simulink model "Check_my_Aerodynamics_for_Mac"  (R2020b)
settings: Solver=FixedStepAuto  StartTime=0.0  StopTime=100  FixedStep=CNT_StepSize  RelTol=1e-3
undefined symbols (not defined in the file): CNT_StepSize
libraries: simulink x2
settings Model: Creator=NicolasS  LastModifiedBy=benjaminh

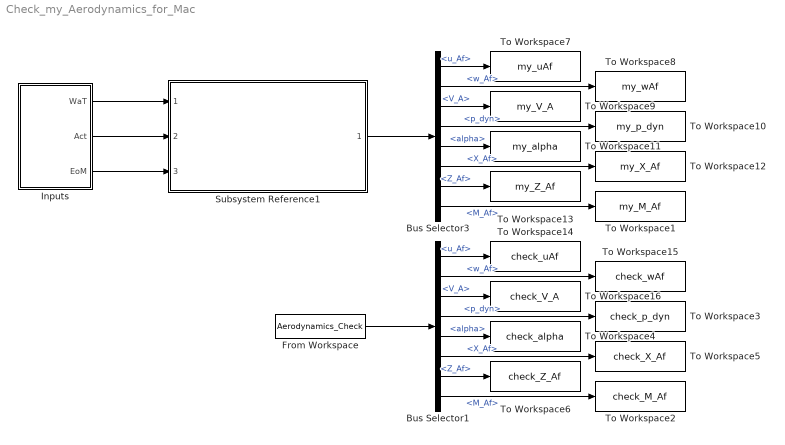
== system Check_my_Aerodynamics_for_Mac ==
  Bus Selector1 : BusSelector  OutputSignals=AirData.u_Af,AirData.w_Af,AirData.V_A,AirData.p_dyn,AirData.alpha,X_Af,Z_Af,M_Af
  Bus Selector3 : BusSelector  OutputSignals=AirData.u_Af,AirData.w_Af,AirData.V_A,AirData.p_dyn,AirData.alpha,X_Af,Z_Af,M_Af
  From Workspace : FromWorkspace  VariableName=Aerodynamics_Check  OutDataTypeStr=Bus: Aero  SampleTime=CNT_StepSize
  Inputs : Subsystem
  Subsystem Reference1 : Subsystem  ReferencedSubsystem=Aerodyn
  To Workspace1 : ToWorkspace  VariableName=my_M_Af  SaveFormat=Timeseries  SampleTime=-1
  To Workspace10 : ToWorkspace  VariableName=my_p_dyn  SaveFormat=Timeseries  SampleTime=-1
  To Workspace11 : ToWorkspace  VariableName=my_alpha  SaveFormat=Timeseries  SampleTime=-1
  To Workspace12 : ToWorkspace  VariableName=my_X_Af  SaveFormat=Timeseries  SampleTime=-1
  To Workspace13 : ToWorkspace  VariableName=my_Z_Af  SaveFormat=Timeseries  SampleTime=-1
  To Workspace14 : ToWorkspace  VariableName=check_uAf  SaveFormat=Timeseries  SampleTime=-1
  To Workspace15 : ToWorkspace  VariableName=check_wAf  SaveFormat=Timeseries  SampleTime=-1
  To Workspace16 : ToWorkspace  VariableName=check_V_A  SaveFormat=Timeseries  SampleTime=-1
  To Workspace2 : ToWorkspace  VariableName=check_M_Af  SaveFormat=Timeseries  SampleTime=-1
  To Workspace3 : ToWorkspace  VariableName=check_p_dyn  SaveFormat=Timeseries  SampleTime=-1
  To Workspace4 : ToWorkspace  VariableName=check_alpha  SaveFormat=Timeseries  SampleTime=-1
  To Workspace5 : ToWorkspace  VariableName=check_X_Af  SaveFormat=Timeseries  SampleTime=-1
  To Workspace6 : ToWorkspace  VariableName=check_Z_Af  SaveFormat=Timeseries  SampleTime=-1
  To Workspace7 : ToWorkspace  VariableName=my_uAf  SaveFormat=Timeseries  SampleTime=-1
  To Workspace8 : ToWorkspace  VariableName=my_wAf  SaveFormat=Timeseries  SampleTime=-1
  To Workspace9 : ToWorkspace  VariableName=my_V_A  SaveFormat=Timeseries  SampleTime=-1
  wires:
  Bus Selector3/7 -> To Workspace13/1  "<Z_Af>"
  Bus Selector3/2 -> To Workspace8/1  "<w_Af>"
  Bus Selector3/6 -> To Workspace12/1  "<X_Af>"
  Bus Selector3/3 -> To Workspace9/1  "<V_A>"
  Bus Selector3/1 -> To Workspace7/1  "<u_Af>"
  Bus Selector3/5 -> To Workspace11/1  "<alpha>"
  Bus Selector3/4 -> To Workspace10/1  "<p_dyn>"
  Subsystem Reference1/1 -> Bus Selector3/1
  Bus Selector3/8 -> To Workspace1/1  "<M_Af>"
  Bus Selector1/4 -> To Workspace3/1  "<p_dyn>"
  Bus Selector1/8 -> To Workspace2/1  "<M_Af>"
  Bus Selector1/7 -> To Workspace6/1  "<Z_Af>"
  Bus Selector1/5 -> To Workspace4/1  "<alpha>"
  Bus Selector1/1 -> To Workspace14/1  "<u_Af>"
  Bus Selector1/6 -> To Workspace5/1  "<X_Af>"
  Bus Selector1/2 -> To Workspace15/1  "<w_Af>"
  Bus Selector1/3 -> To Workspace16/1  "<V_A>"
  Inputs/2(Act) -> Subsystem Reference1/2
  Inputs/1(WaT) -> Subsystem Reference1/1
  Inputs/3(EoM) -> Subsystem Reference1/3
  From Workspace/1 -> Bus Selector1/1

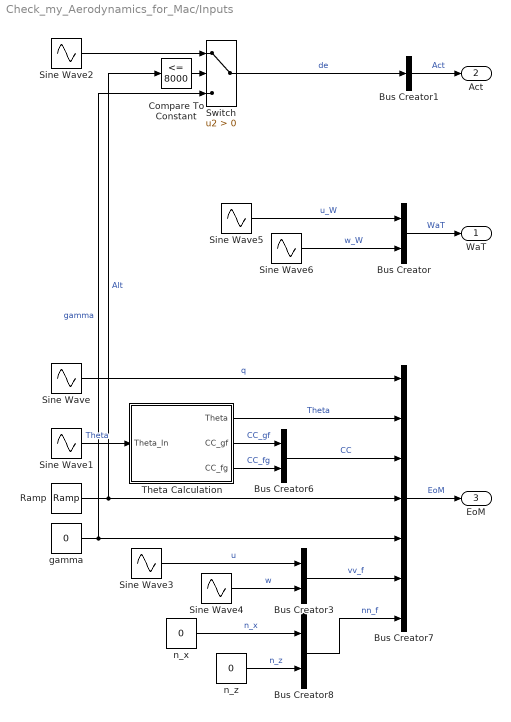
== system Check_my_Aerodynamics_for_Mac/Inputs ==
  Bus Creator : BusCreator  Inputs=2  OutDataTypeStr=Bus: WaT
  Bus Creator1 : BusCreator  Inputs=1  OutDataTypeStr=Bus: Act
  Bus Creator3 : BusCreator  Inputs=2  OutDataTypeStr=Bus: vv_f
  Bus Creator6 : BusCreator  Inputs=2  OutDataTypeStr=Bus: CC
  Bus Creator7 : BusCreator  Inputs=7  OutDataTypeStr=Bus: EoM
  Bus Creator8 : BusCreator  Inputs=2  OutDataTypeStr=Bus: nn_f
  Compare To Constant : simulink/Logic and Bit Operations/Compare To Constant  relop=<=  const=8000  OutDataTypeStr=boolean
  Ramp : simulink/Sources/Ramp  slope=-50  start=0  InitialOutput=10000
  Sine Wave : Sin  Amplitude=0.05  Frequency=0.9  SampleTime=CNT_StepSize
  Sine Wave1 : Sin  Amplitude=0.1  Frequency=0.1  Phase=-45  SampleTime=CNT_StepSize
  Sine Wave2 : Sin  Amplitude=0.03  Frequency=1.3  Phase=-67  SampleTime=CNT_StepSize
  Sine Wave3 : Sin  Amplitude=20  Bias=140  Frequency=0.1  Phase=34  SampleTime=CNT_StepSize
  Sine Wave4 : Sin  Amplitude=5  Bias=7  Frequency=0.24  SampleTime=CNT_StepSize
  Sine Wave5 : Sin  Amplitude=15  Frequency=2*pi/40  Phase=63  SampleTime=CNT_StepSize
  Sine Wave6 : Sin  Amplitude=5  Frequency=2*pi/40  Phase=-15  SampleTime=CNT_StepSize
  Switch : Switch  Criteria=u2 > Threshold
  Theta Calculation : MATLAB Function  TreatAsAtomicUnit=on
  gamma : Constant  Value=0  SampleTime=-1
  n_x : Constant  Value=0  SampleTime=-1
  n_z : Constant  Value=0  SampleTime=-1
  WaT : Outport  OutDataTypeStr=Bus: WaT
  Act : Outport  Port=2  OutDataTypeStr=Bus: Act
  EoM : Outport  Port=3  OutDataTypeStr=Bus: EoM
  wires:
  Bus Creator8/1 -> Bus Creator7/7  "nn_f"
  Sine Wave3/1 -> Bus Creator3/1  "u"
  n_x/1 -> Bus Creator8/1  "n_x"
  Bus Creator3/1 -> Bus Creator7/6  "vv_f"
  Sine Wave5/1 -> Bus Creator/1  "u_W"
  Theta Calculation/2(CC_gf) -> Bus Creator6/1  "CC_gf"
  Bus Creator/1 -> WaT/1  "WaT"
  n_z/1 -> Bus Creator8/2  "n_z"
  Ramp/1 -> Bus Creator7/4, Compare To Constant/1  "Alt"
  Sine Wave2/1 -> Switch/1
  Compare To Constant/1 -> Switch/2
  Bus Creator6/1 -> Bus Creator7/3  "CC"
  Sine Wave4/1 -> Bus Creator3/2  "w"
  Switch/1 -> Bus Creator1/1  "de"
  gamma/1 -> Switch/3, Bus Creator7/5  "gamma"
  Bus Creator1/1 -> Act/1  "Act"
  Sine Wave/1 -> Bus Creator7/1  "q"
  Theta Calculation/3(CC_fg) -> Bus Creator6/2  "CC_fg"
  Theta Calculation/1(Theta) -> Bus Creator7/2  "Theta"
  Sine Wave1/1 -> Theta Calculation/1(Theta_In)  "Theta"
  Bus Creator7/1 -> EoM/1  "EoM"
  Sine Wave6/1 -> Bus Creator/2  "w_W"

== matlab function Check_my_Aerodynamics_for_Mac/Inputs/Theta Calculation ==
  data: Theta output size=1; CC_gf output size=[2 2]; CC_fg output size=[2 2]; Theta_In input size=1
function [Theta,CC_gf,CC_fg] = fcn(Theta_In)

Theta = mod(Theta_In+pi,2*pi)-pi; % pi bound

CC_fg = [cos(Theta)  -sin(Theta);
         sin(Theta)   cos(Theta)];
     
CC_gf = CC_fg';
